simulink model "Led_Switch"  (R2016a)
settings: Solver=FixedStepDiscrete  StartTime=0.0  StopTime=10.0  RelTol=1e-3
libraries: simulink x1
settings Model: Creator=Mohamed Fawzy  LastModifiedBy=Mohamed Fawzy
settings OptimizationCC: DefaultParameterBehavior=Inlined  OptimizeModelRefInitCode=on  LifeSpan=1
settings RTWCC: SystemTargetFile=ert.tlc  GenCodeOnly=on  GenerateMakefile=off  TemplateMakefile=ert_default_tmf  GenerateReport=on  IncludeHyperlinkInReport=on  LaunchReport=on  GenerateTraceInfo=on  GenerateTraceReport=on  GenerateTraceReportSl=on  GenerateTraceReportSf=on  GenerateTraceReportEml=on
settings CodeAppCC: ForceParamTrailComments=on  IgnoreCustomStorageClasses=off  OperatorAnnotations=on  SimulinkDataObjDesc=on  SFDataObjDesc=on  MATLABFcnDesc=on  InsertBlockDesc=on  MATLABSourceComments=on
settings ERTTargetCC: GenerateSampleERTMain=on  SuppressErrorStatus=on  InlinedParameterPlacement=NonHierarchical  ERTCustomFileTemplate=example_file_process.tlc

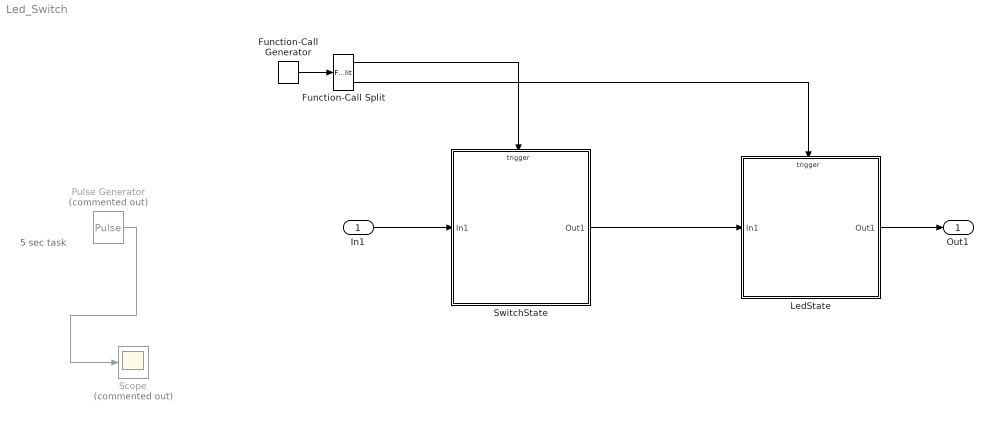
== system Led_Switch ==
  note: 5 sec task
  In1 : Inport  OutDataTypeStr=uint8
  Function-Call Generator : simulink/Ports & Subsystems/Function-Call Generator  sample_time=1  numberOfIterations=1
  Function-Call Split : FunctionCallSplit  IconShape=distinctive  NumOutputPorts=2  OutputPortLayout=default
  LedState : Subsystem  TreatAsAtomicUnit=on
  Pulse Generator : DiscretePulseGenerator  Commented=on  PulseType=Time based  Period=5
  Scope : Scope  Commented=on
  SwitchState : Subsystem  TreatAsAtomicUnit=on
  Out1 : Outport  OutDataTypeStr=uint8
  wires:
  Function-Call Generator/1 -> Function-Call Split/1
  Function-Call Split/1 -> SwitchState/Trigger
  Function-Call Split/2 -> LedState/Trigger
  Pulse Generator/1 -> Scope/1
  SwitchState/1(Out1) -> LedState/1(In1)
  In1/1 -> SwitchState/1(In1)
  LedState/1(Out1) -> Out1/1

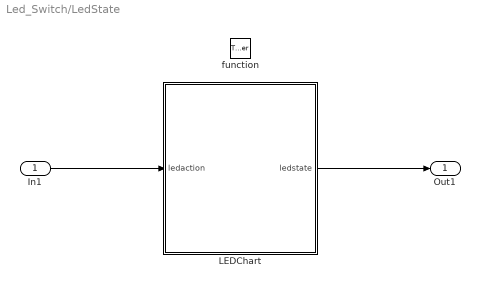
== system Led_Switch/LedState ==
  In1 : Inport  OutDataTypeStr=uint8
  function : TriggerPort  TriggerType=function-call  VariantControl=Variant  StatesWhenEnabling=reset
  LEDChart : Stateflow chart  TreatAsAtomicUnit=on
  Out1 : Outport  OutDataTypeStr=uint8
  wires:
  In1/1 -> LEDChart/1(ledaction)
  LEDChart/1(ledstate) -> Out1/1

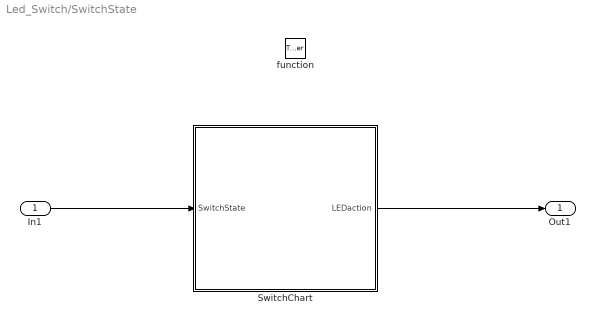
== system Led_Switch/SwitchState ==
  In1 : Inport  OutDataTypeStr=uint8
  function : TriggerPort  TriggerType=function-call  VariantControl=Variant  StatesWhenEnabling=reset
  SwitchChart : Stateflow chart  TreatAsAtomicUnit=on
  Out1 : Outport  OutDataTypeStr=uint8
  wires:
  In1/1 -> SwitchChart/1(SwitchState)
  SwitchChart/1(LEDaction) -> Out1/1

== stateflow chart Led_Switch/LedState/LEDChart ==
  state Led_Normal
    state LedOff
      en:
      ledstate= uint8(0);
    state LedOn
      en:
      ledstate=1;
    (default) -> LedOff
    LedOn -> LedOff : [ledaction==0]
    LedOff -> LedOn : [ledaction==1]
  state Led_Fault
  (default) -> Led_Normal
  data: ledaction input uint8; ledstate output uint8

== stateflow chart Led_Switch/SwitchState/SwitchChart ==
  state Sw_Normal
    state NotPressed
      en:
      LEDaction= uint8(0);
    state Pressed
      en:
      LEDaction=uint8(1);
    (default) -> NotPressed
    Pressed -> NotPressed : [SwitchState==0]
    NotPressed -> Pressed : [SwitchState==1]
  (default) -> Sw_Normal
  data: SwitchState input uint8; LEDaction output uint8
